simulink model "simulation"  (R2018a)
settings: Solver=VariableStepAuto  StartTime=0.0  StopTime=10.0  RelTol=1e-3
undefined symbols (not defined in the file or in its folder): booleanControl, difuseControl
settings Model: Creator=daniel  LastModifiedBy=daniel

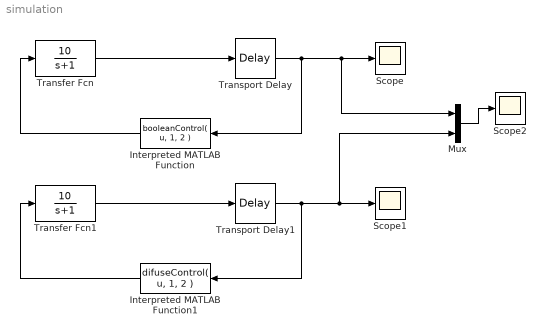
== system simulation ==
  Interpreted MATLAB Function : MATLABFcn  MATLABFcn=booleanControl( u, 1, 2 )
  Interpreted MATLAB Function1 : MATLABFcn  MATLABFcn=difuseControl( u, 1, 2 )
  Mux : Mux  Inputs=2
  Scope : Scope
  Scope1 : Scope
  Scope2 : Scope
  Transfer Fcn : TransferFcn  Numerator=[10]  Denominator=[1 1]
  Transfer Fcn1 : TransferFcn  Numerator=[10]  Denominator=[1 1]
  Transport Delay : TransportDelay
  Transport Delay1 : TransportDelay
  wires:
  Interpreted MATLAB Function/1 -> Transfer Fcn/1
  Transfer Fcn/1 -> Transport Delay/1
  Transport Delay/1 -> Interpreted MATLAB Function/1, Mux/1, Scope/1
  Transfer Fcn1/1 -> Transport Delay1/1
  Transport Delay1/1 -> Interpreted MATLAB Function1/1, Mux/2, Scope1/1
  Interpreted MATLAB Function1/1 -> Transfer Fcn1/1
  Mux/1 -> Scope2/1
